simulink model "SynchronouslChange0"  (R2017b)
settings: Solver=ode23tb  StartTime=0.0  StopTime=0.5  MaxStep=1e-4  RelTol=1e-3
libraries: powerlib x7, simulink x1
settings Model: Creator=80573  LastModifiedBy=80573

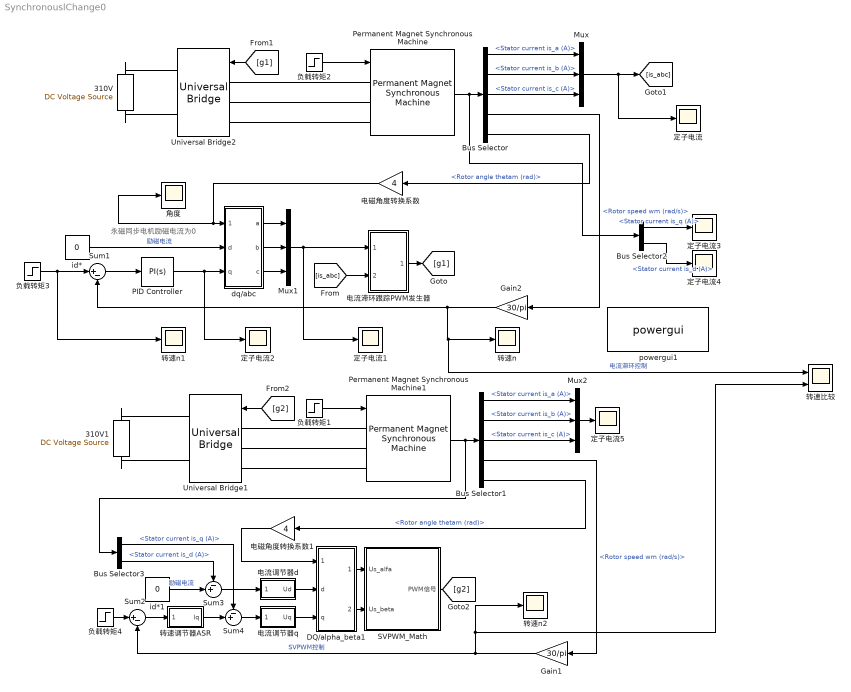
== system SynchronouslChange0 ==
  note: 永磁同步电机励磁电流为0
  310V : powerlib/Electrical Sources/DC Voltage Source  Amplitude=310  Measurements=None
  310V1 : powerlib/Electrical Sources/DC Voltage Source  Amplitude=310  Measurements=None
  Bus Selector : BusSelector  OutputSignals=Stator current is_a (A),Stator current is_b (A),Stator current is_c (A),Rotor speed wm (rad/s),Rotor angle thetam (rad)
  Bus Selector1 : BusSelector  OutputSignals=Stator current is_a (A),Stator current is_b (A),Stator current is_c (A),Rotor speed wm (rad/s),Rotor angle thetam (rad)
  Bus Selector2 : BusSelector  OutputSignals=Stator current is_q (A),Stator current is_d (A)
  Bus Selector3 : BusSelector  OutputSignals=Stator current is_q (A),Stator current is_d (A)
  DQ/alpha_beta1 : Subsystem
  Gain1 : Gain  Gain=30/pi
  Gain2 : Gain  Gain=30/pi
  Mux : Mux  Inputs=3
  Mux1 : Mux  Inputs=3
  Mux2 : Mux  Inputs=3
  PID Controller : simulink/Continuous/PID Controller  Controller=PI  TimeDomain=Continuous-time  SampleTime=-1  IntegratorMethod=Forward Euler  FilterMethod=Forward Euler  Form=Parallel  UseFilter=on  ControllerParametersSource=internal  P=0.05  I=8  D=0  N=100  InitialConditionSource=internal  InitialConditionForIntegrator=0  InitialConditionForFilter=0  ExternalReset=none  LimitOutput=on  UpperSaturationLimit=200  LowerSaturationLimit=-inf  LinearizeAsGain=on  AntiWindupMode=none  Kb=1  TrackingMode=off  Kt=1  PParamMin=[]  PParamMax=[]  IParamMin=[]  IParamMax=[]  DParamMin=[]  DParamMax=[]  NParamMin=[]  NParamMax=[]  KbParamMin=[]  KbParamMax=[]  KtParamMin=[]  KtParamMax=[]  POutMin=[]  POutMax=[]  IOutMin=[]  IOutMax=[]  DOutMin=[]  DOutMax=[]  NOutMin=[]  NOutMax=[]  KbOutMin=[]  KbOutMax=[]  KtOutMin=[]  KtOutMax=[]  IntegratorOutMin=[]  IntegratorOutMax=[]  FilterOutMin=[]  FilterOutMax=[]  SumOutMin=[]  SumOutMax=[]  SumI1OutMin=[]  SumI1OutMax=[]  SumI2OutMin=[]  SumI2OutMax=[]  SumI3OutMin=[]  SumI3OutMax=[]  SumDOutMin=[]  SumDOutMax=[]  SaturationOutMin=[]  SaturationOutMax=[]  IntegratorContinuousStateAttributes=''  IntegratorStateMustResolveToSignalObject=off  IntegratorRTWStateStorageClass=Auto  FilterContinuousStateAttributes=''  FilterStateMustResolveToSignalObject=off  FilterRTWStateStorageClass=Auto  DifferentiatorICPrevScaledInput=0  DifferentiatorOutMin=[]  DifferentiatorOutMax=[]  InitialConditionSetting=State (most efficient)  FilterDiffOutCoefMin=[]  FilterDiffOutCoefMax=[]  SumDenOutMin=[]  SumDenOutMax=[]  SumNumOutMin=[]  SumNumOutMax=[]  ReciprocalOutMin=[]  ReciprocalOutMax=[]  DivideOutMin=[]  DivideOutMax=[]  TunerSelectOption=Transfer Function Based (PID Tuner App)
  Permanent Magnet Synchronous Machine : powerlib/Machines/Permanent Magnet Synchronous Machine  NbPhases=3  FluxDistribution=Sinusoidal  RotorType=Salient-pole  MechanicalLoad=Torque Tm  PresetModel=No  ShowDetailedParameters=on  MeasurementBus=off  Resistance=2.785  Inductance=8.5e-3  dqInductances=[0.0085 0.0085]  La=0.02682  MachineConstant=Flux linkage established by magnets (V.s)  Flux=0.175  VoltageCst=126.966  TorqueCst=1.05  Flat=120  Mechanical=[0.001 0.008 4 0]  PolePairs=2  InitialConditions=[0,0, 0,0]  InitialConditions5ph=[0 0 0 0 0 0]  TsPowergui=0  TsBlock=-1  RefAngle=Aligned with phase A axis (original Park)
      settings: SourceProductName=Simscape Power Systems
  Permanent Magnet Synchronous Machine1 : powerlib/Machines/Permanent Magnet Synchronous Machine  NbPhases=3  FluxDistribution=Sinusoidal  RotorType=Salient-pole  MechanicalLoad=Torque Tm  PresetModel=No  ShowDetailedParameters=on  MeasurementBus=off  Resistance=2.785  Inductance=8.5e-3  dqInductances=[0.0085 0.0085]  La=0.02682  MachineConstant=Flux linkage established by magnets (V.s)  Flux=0.175  VoltageCst=126.966  TorqueCst=1.05  Flat=120  Mechanical=[0.001 0.008 4 0]  PolePairs=2  InitialConditions=[0,0, 0,0]  InitialConditions5ph=[0 0 0 0 0 0]  TsPowergui=0  TsBlock=-1  RefAngle=Aligned with phase A axis (original Park)
      settings: SourceProductName=Simscape Power Systems
  SVPWM_Math : Subsystem
  Sum1 : Sum  Inputs=|+-
  Sum2 : Sum  Inputs=|+-
  Sum3 : Sum  Inputs=-+|
  Sum4 : Sum  Inputs=-+|
  Universal Bridge1 : powerlib/Power Electronics/Universal Bridge  Arms=3  SnubberResistance=1e5  SnubberCapacitance=inf  Device=IGBT / Diodes  Ron=1e-3  Lon=0  ForwardVoltages="[  0  0  ]"  ForwardVoltage=0  GTOparameters=[ 10e-6 , 20e-6 ]  IGBTparameters=[ 1e-6 , 2e-6 ]  Measurements=None  Measurements_2=None  converterType=Rectifier
  Universal Bridge2 : powerlib/Power Electronics/Universal Bridge  Arms=3  SnubberResistance=1e5  SnubberCapacitance=inf  Device=IGBT / Diodes  Ron=1e-3  Lon=0  ForwardVoltages="[  0  0  ]"  ForwardVoltage=0  GTOparameters=[ 10e-6 , 20e-6 ]  IGBTparameters=[ 1e-6 , 2e-6 ]  Measurements=None  Measurements_2=None  converterType=Rectifier
  dq/abc : Subsystem
  id* : Constant  Value=0
  id*1 : Constant  Value=0
  powergui1 : powerlib/powergui  SimulationMode=Discrete  SampleTime=1e-6  frequency=50  Iterations=50  frequencyindice=0  Pbase=100e6  ErrMax=1e-4  UnitsV=kV  UnitsW=MW  buscounter=0  FunctionMessages=off  echomessages=off  EnableUseOfTLC=off  CurrentSourceSwitches=off  DisableSnubberDevices=off  DisableRonSwitches=off  DisableVfSwitches=off  DisplayEquations=off  SolverType=Tustin/Backward Euler (TBE)  Interpol=off  ExternalGateDelay=off  methode=off  Ts=100  x0status=zero  SPID=on  SwTol=0  HookPort=off  RestoreLinks=warning  ResistiveCurrentMeasurement=off  Frange=[0:2:500]  Ylog=off  Xlog=on  ShowGrid=off  save=off  variable=ZData  structure=0  ZoomFFT=on  StartTime=0.0  cycles=1  DisplayStyle=1  fundamental=60  FreqAxis=off  MaxFrequency=1000  frequencyindicesteady=1  RmsSteady=1  display=off
  定子电流{,1..5} (6 alike) : Scope
  电流滞环跟踪PWM发生器 : Subsystem
  电流调节器d : Subsystem
  电流调节器q : Subsystem
  电磁角度转换系数 : Gain  Gain=4
  电磁角度转换系数1 : Gain  Gain=4
  角度 : Scope
  负载转矩1 : Step  Time=0.2  Before=10  After=20  SampleTime=0
  负载转矩2 : Step  Time=0.2  Before=10  After=20  SampleTime=0
  负载转矩3 : Step  Time=0.3  Before=1000  After=1200  SampleTime=0
  负载转矩4 : Step  Time=0.3  Before=1000  After=1200  SampleTime=0
  转速n : Scope
  转速n1 : Scope
  转速n2 : Scope
  转速比较 : Scope  NumInputPorts=2
  转速调节器ASR : Subsystem
  wires:
  转速调节器ASR/1(Iq) -> Sum4/2
  id*/1 -> dq/abc/2(d)  "励磁电流"
  负载转矩1/1 -> Permanent Magnet Synchronous Machine1/1
  DQ/alpha_beta1/2(beta) -> SVPWM_Math/2(Us_beta)
  Bus Selector1/1 -> Mux2/1  "<Stator current is_a (A)>"
  Bus Selector1/2 -> Mux2/2  "<Stator current is_b (A)>"
  负载转矩4/1 -> Sum2/1
  电流调节器q/1(Uq) -> DQ/alpha_beta1/3(q)
  Gain1/1 -> Sum2/2, 转速比较/2, 转速n2/1  "SVPWM控制"
  Mux2/1 -> 定子电流5/1
  Permanent Magnet Synchronous Machine1/1 -> Bus Selector3/1, Bus Selector1/1
  Bus Selector3/2 -> Sum3/1  "<Stator current is_d (A)>"
  Bus Selector1/5 -> 电磁角度转换系数1/1  "<Rotor angle thetam (rad)>"
  Bus Selector2/2 -> 定子电流4/1  "<Stator current is_d (A)>"
  [g2] -> Universal Bridge1/1
  Bus Selector1/4 -> Gain1/1  "<Rotor speed wm (rad/s)>"
  Sum1/1 -> PID Controller/1
  电磁角度转换系数1/1 -> DQ/alpha_beta1/1(theta)
  Sum2/1 -> 转速调节器ASR/1("  ")
  dq/abc/2(b) -> Mux1/2
  Sum4/1 -> 电流调节器q/1("  ")
  id*1/1 -> Sum3/2  "励磁电流"
  [g1] -> Universal Bridge2/1
  电磁角度转换系数/1 -> 角度/1, dq/abc/1(theta)
  负载转矩2/1 -> Permanent Magnet Synchronous Machine/1
  Bus Selector/2 -> Mux/2  "<Stator current is_b (A)>"
  Bus Selector/3 -> Mux/3  "<Stator current is_c (A)>"
  Bus Selector3/1 -> Sum4/1  "<Stator current is_q (A)>"
  dq/abc/1(a) -> Mux1/1
  Bus Selector/5 -> 电磁角度转换系数/1  "<Rotor angle thetam (rad)>"
  负载转矩3/1 -> 转速n1/1, Sum1/1
  Permanent Magnet Synchronous Machine/1 -> Bus Selector2/1, Bus Selector/1
  Bus Selector/1 -> Mux/1  "<Stator current is_a (A)>"
  电流调节器d/1(Ud) -> DQ/alpha_beta1/2(d)
  Bus Selector2/1 -> 定子电流3/1  "<Stator current is_q (A)>"
  Bus Selector1/3 -> Mux2/3  "<Stator current is_c (A)>"
  Gain2/1 -> Sum1/2, 转速比较/1, 转速n/1  "电流滞环控制"
  DQ/alpha_beta1/1(alpha) -> SVPWM_Math/1(Us_alfa)
  [is_abc] -> 电流滞环跟踪PWM发生器/2(Iabc)
  Mux1/1 -> 电流滞环跟踪PWM发生器/1(Iabc*), 定子电流1/1
  Bus Selector/4 -> Gain2/1  "<Rotor speed wm (rad/s)>"
  Sum3/1 -> 电流调节器d/1("  ")
  dq/abc/3(c) -> Mux1/3
  Mux/1 -> 定子电流/1, [is_abc]
  SVPWM_Math/1(PWM信号) -> [g2]
  PID Controller/1 -> 定子电流2/1, dq/abc/3(q)
  电流滞环跟踪PWM发生器/1(pulse) -> [g1]
  connections:
  Universal Bridge1/LConn3 -- Permanent Magnet Synchronous Machine1/LConn3
  Universal Bridge2/LConn1 -- Permanent Magnet Synchronous Machine/LConn1
  310V/RConn1 -- Universal Bridge2/RConn1
  Universal Bridge2/LConn3 -- Permanent Magnet Synchronous Machine/LConn3
  Universal Bridge1/LConn1 -- Permanent Magnet Synchronous Machine1/LConn1
  310V/LConn1 -- Universal Bridge2/RConn2
  310V1/LConn1 -- Universal Bridge1/RConn2
  Universal Bridge1/LConn2 -- Permanent Magnet Synchronous Machine1/LConn2
  Universal Bridge2/LConn2 -- Permanent Magnet Synchronous Machine/LConn2
  310V1/RConn1 -- Universal Bridge1/RConn1

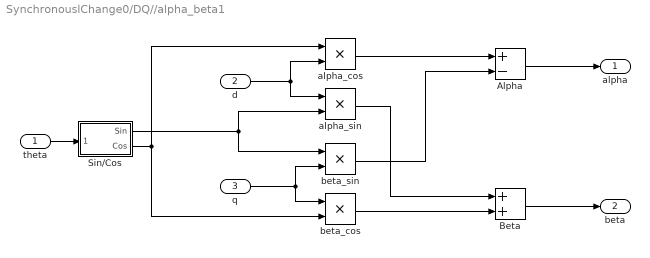
== system SynchronouslChange0/DQ//alpha_beta1 ==
  theta : Inport
  d : Inport  Port=2
  q : Inport  Port=3
  Alpha : Sum  Inputs=+-
  Beta : Sum
  Sin/Cos : Subsystem
  alpha_cos : Product
  alpha_sin : Product
  beta_cos : Product
  beta_sin : Product
  alpha : Outport
  beta : Outport  Port=2
  wires:
  Sin/Cos/2(Cos) -> beta_cos/2, alpha_cos/1
  q/1 -> beta_sin/2, beta_cos/1
  Sin/Cos/1(Sin) -> beta_sin/1, alpha_sin/2
  alpha_sin/1 -> Beta/1
  theta/1 -> Sin/Cos/1(theta)
  beta_sin/1 -> Alpha/2
  beta_cos/1 -> Beta/2
  Alpha/1 -> alpha/1
  alpha_cos/1 -> Alpha/1
  d/1 -> alpha_cos/2, alpha_sin/1
  Beta/1 -> beta/1

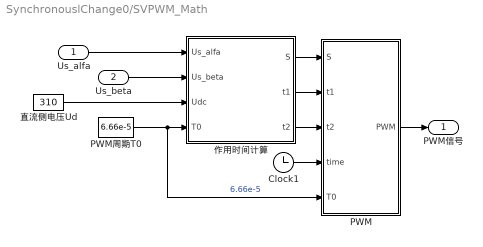
== system SynchronouslChange0/SVPWM_Math ==
  Us_alfa : Inport
  Us_beta : Inport  Port=2
  Clock1 : Clock
  PWM : MATLAB Function  TreatAsAtomicUnit=on
  PWM周期T0 : Constant  Value=6.66e-5
  作用时间计算 : MATLAB Function  TreatAsAtomicUnit=on
  直流侧电压Ud : Constant  Value=310
  PWM信号 : Outport
  wires:
  作用时间计算/2(t1) -> PWM/2(t1)
  作用时间计算/3(t2) -> PWM/3(t2)
  PWM/1(PWM) -> PWM信号/1
  Us_alfa/1 -> 作用时间计算/1(Us_alfa)
  Us_beta/1 -> 作用时间计算/2(Us_beta)
  直流侧电压Ud/1 -> 作用时间计算/3(Udc)
  PWM周期T0/1 -> PWM/5(T0), 作用时间计算/4(T0)  "6.66e-5"
  Clock1/1 -> PWM/4(time)
  作用时间计算/1(S) -> PWM/1(S)

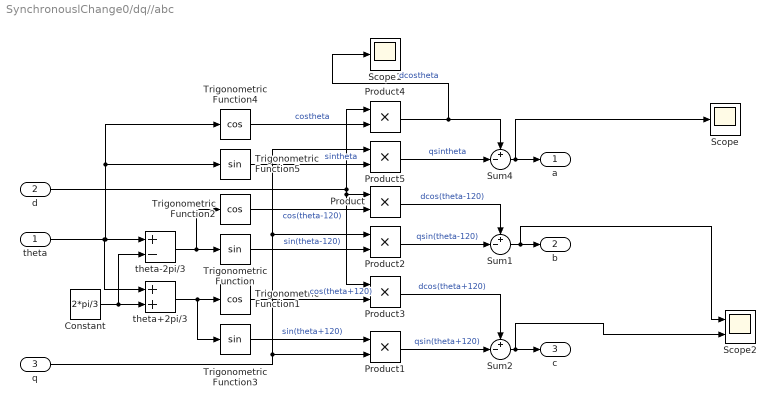
== system SynchronouslChange0/dq//abc ==
  theta : Inport
  d : Inport  Port=2
  q : Inport  Port=3
  Constant : Constant  Value=2*pi/3
  Product{,1..5} (6 alike) : Product
  Scope : Scope
  Scope1 : Scope
  Scope2 : Scope  NumInputPorts=2
  Sum1 : Sum  Inputs=+-|
  Sum2 : Sum  Inputs=+-|
  Sum4 : Sum  Inputs=+-|
  Trigonometric Function : Trigonometry
  Trigonometric Function1 : Trigonometry  Operator=cos
  Trigonometric Function2 : Trigonometry  Operator=cos
  Trigonometric Function3 : Trigonometry
  Trigonometric Function4 : Trigonometry  Operator=cos
  Trigonometric Function5 : Trigonometry
  theta+2pi/3 : Sum
  theta-2pi/3 : Sum  Inputs=+-
  a : Outport
  b : Outport  Port=2
  c : Outport  Port=3
  wires:
  Trigonometric Function5/1 -> Product5/2  "sintheta"
  Product/1 -> Sum1/1  "dcos(theta-120)"
  Trigonometric Function1/1 -> Product3/2  "cos(theta+120)"
  Product3/1 -> Sum2/1  "dcos(theta+120)"
  d/1 -> Product/1, Product3/1, Product4/1
  Constant/1 -> theta+2pi/3/2, theta-2pi/3/2
  theta/1 -> Trigonometric Function4/1, Trigonometric Function5/1, theta-2pi/3/1, theta+2pi/3/1
  theta+2pi/3/1 -> Trigonometric Function3/1, Trigonometric Function1/1
  q/1 -> Product5/1, Product2/1, Product1/2
  Trigonometric Function/1 -> Product2/2  "sin(theta-120)"
  Product4/1 -> Scope1/1, Sum4/1  "dcostheta"
  Product5/1 -> Sum4/2  "qsintheta"
  theta-2pi/3/1 -> Trigonometric Function2/1, Trigonometric Function/1
  Product1/1 -> Sum2/2  "qsin(theta+120)"
  Trigonometric Function2/1 -> Product/2  "cos(theta-120)"
  Sum4/1 -> Scope/1, a/1
  Sum1/1 -> Scope2/1, b/1
  Trigonometric Function4/1 -> Product4/2  "costheta"
  Trigonometric Function3/1 -> Product1/1  "sin(theta+120)"
  Product2/1 -> Sum1/2  "qsin(theta-120)"
  Sum2/1 -> Scope2/2, c/1

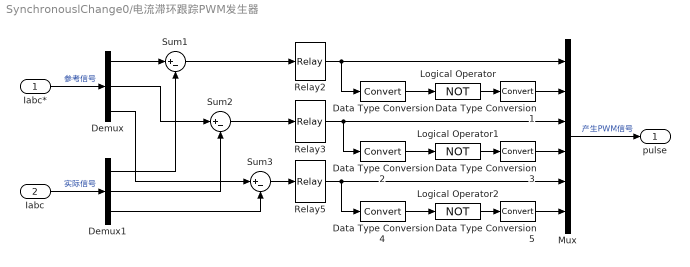
== system SynchronouslChange0/电流滞环跟踪PWM发生器 ==
  Iabc* : Inport
  Iabc : Inport  Port=2
  Data Type Conversion{,1..5} (6 alike) : DataTypeConversion
  Demux : Demux  Outputs=3
  Demux1 : Demux  Outputs=3
  Logical Operator : Logic  Operator=NOT  Inputs=1  AllPortsSameDT=off
  Logical Operator1 : Logic  Operator=NOT  Inputs=1  AllPortsSameDT=off
  Logical Operator2 : Logic  Operator=NOT  Inputs=1  AllPortsSameDT=off
  Mux : Mux  Inputs=6
  Relay2 : Relay  OnSwitchValue=0.1  OffSwitchValue=-0.1  ZeroCross=off
  Relay3 : Relay  OnSwitchValue=0.1  OffSwitchValue=-0.1  ZeroCross=off
  Relay5 : Relay  OnSwitchValue=0.1  OffSwitchValue=-0.1  ZeroCross=off
  Sum1 : Sum  Inputs=|+-
  Sum2 : Sum  Inputs=|+-
  Sum3 : Sum  Inputs=|+-
  pulse : Outport
  wires:
  Relay2/1 -> Data Type Conversion/1, Mux/1
  Data Type Conversion/1 -> Logical Operator/1
  Logical Operator/1 -> Data Type Conversion1/1
  Data Type Conversion1/1 -> Mux/2
  Mux/1 -> pulse/1  "产生PWM信号"
  Sum1/1 -> Relay2/1
  Demux/1 -> Sum1/1
  Demux1/3 -> Sum3/2
  Iabc/1 -> Demux1/1  "实际信号"
  Iabc*/1 -> Demux/1  "参考信号"
  Sum2/1 -> Relay3/1
  Logical Operator1/1 -> Data Type Conversion3/1
  Data Type Conversion3/1 -> Mux/4
  Data Type Conversion2/1 -> Logical Operator1/1
  Relay3/1 -> Data Type Conversion2/1, Mux/3
  Logical Operator2/1 -> Data Type Conversion5/1
  Data Type Conversion5/1 -> Mux/6
  Data Type Conversion4/1 -> Logical Operator2/1
  Relay5/1 -> Data Type Conversion4/1, Mux/5
  Sum3/1 -> Relay5/1
  Demux/2 -> Sum2/1
  Demux1/1 -> Sum1/2
  Demux1/2 -> Sum2/2
  Demux/3 -> Sum3/1

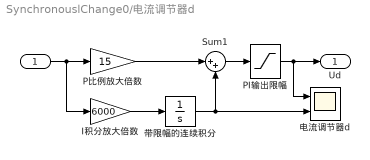
== system SynchronouslChange0/电流调节器d ==
  "  " : Inport
  I积分放大倍数 : Gain  Gain=6000
  PI输出限幅 : Saturate  UpperLimit=400  LowerLimit=-400
  P比例放大倍数 : Gain  Gain=15
  Sum1 : Sum  Inputs=|++
  带限幅的连续积分 : Integrator  UpperSaturationLimit=30  LowerSaturationLimit=-30
  电流调节器d : Scope  NumInputPorts=2
  Ud : Outport
  wires:
  Sum1/1 -> PI输出限幅/1
  PI输出限幅/1 -> 电流调节器d/1, Ud/1
  P比例放大倍数/1 -> Sum1/1
  I积分放大倍数/1 -> 带限幅的连续积分/1
  带限幅的连续积分/1 -> 电流调节器d/2, Sum1/2
  "  "/1 -> I积分放大倍数/1, P比例放大倍数/1

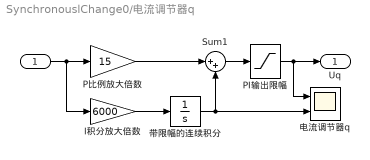
== system SynchronouslChange0/电流调节器q ==
  "  " : Inport
  I积分放大倍数 : Gain  Gain=6000
  PI输出限幅 : Saturate  UpperLimit=300  LowerLimit=-300
  P比例放大倍数 : Gain  Gain=15
  Sum1 : Sum  Inputs=|++
  带限幅的连续积分 : Integrator  LimitOutput=on  UpperSaturationLimit=400  LowerSaturationLimit=-400
  电流调节器q : Scope  NumInputPorts=2
  Uq : Outport
  wires:
  Sum1/1 -> PI输出限幅/1
  PI输出限幅/1 -> 电流调节器q/1, Uq/1
  P比例放大倍数/1 -> Sum1/1
  I积分放大倍数/1 -> 带限幅的连续积分/1
  带限幅的连续积分/1 -> 电流调节器q/2, Sum1/2
  "  "/1 -> I积分放大倍数/1, P比例放大倍数/1

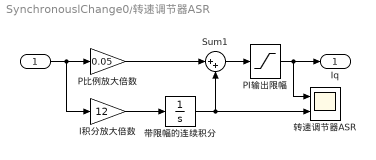
== system SynchronouslChange0/转速调节器ASR ==
  "  " : Inport
  I积分放大倍数 : Gain  Gain=12
  PI输出限幅 : Saturate  UpperLimit=25  LowerLimit=-25
  P比例放大倍数 : Gain  Gain=0.05
  Sum1 : Sum  Inputs=|++
  带限幅的连续积分 : Integrator  LimitOutput=on  UpperSaturationLimit=30  LowerSaturationLimit=-30
  转速调节器ASR : Scope  NumInputPorts=2
  Iq : Outport
  wires:
  Sum1/1 -> PI输出限幅/1
  PI输出限幅/1 -> 转速调节器ASR/1, Iq/1
  P比例放大倍数/1 -> Sum1/1
  I积分放大倍数/1 -> 带限幅的连续积分/1
  带限幅的连续积分/1 -> 转速调节器ASR/2, Sum1/2
  "  "/1 -> I积分放大倍数/1, P比例放大倍数/1

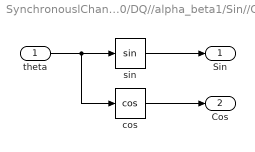
== system SynchronouslChange0/DQ//alpha_beta1/Sin//Cos ==
  theta : Inport
  cos : Trigonometry  Operator=cos
  sin : Trigonometry
  Sin : Outport
  Cos : Outport  Port=2
  wires:
  sin/1 -> Sin/1
  theta/1 -> sin/1, cos/1
  cos/1 -> Cos/1

== matlab function SynchronouslChange0/SVPWM_Math/作用时间计算 ==
  data: Us_alfa input; S output; Us_beta input; Udc input; T0 input; t1 output; t2 output
function [S,t1,t2] = fcn(Us_alfa,Us_beta,Udc,T0)
% This block supports an embeddable subset of the MATLAB language.
% See the help menu for details.
%--------------------为了方便推导作用时间做出的设定值------------------------
X=sqrt(3)*T0*Us_beta/Udc;                           
Y=sqrt(3)/2*T0*Us_beta/Udc+3/2*T0*Us_alfa/Udc;     
Z=sqrt(3)/2*T0*Us_beta/Udc-3/2*T0*Us_alfa/Udc;      
%--------------------------------扇区值判断---------------------------------
%Uref1*sqrt(3)
%(Uref1+Uref2)*sqrt(3)
%(Uref1+Uref3)*sqrt(3)
%--------------------------------------------------------------------------
if(Us_beta>0)                                       %Uref1>0
    A=1;
else
    A=0;
end                                                                                                                                                                                                                                                                                                                                                                                                                                                                                                                                                                                                                                                                                                                                                                                                                                                                                                                                                                                                                                                                                                                                                                                                                                                                                   
if((sqrt(3)*Us_alfa-Us_beta)>0)                     %Uref2>0
    B=1;
else
    B=0; 
end
if((-sqrt(3)*Us_alfa-Us_beta)>0)                    %%Uref3>0
    C=1;
else
    C=0;
end
N=A+2*B+4*C;                                        %扇区值N，而不是扇区编号！！！！！！！
%--------------------------------------------------------------------------
%-----------------------------------分割线----------------------------------

%-----------------------------矢量作用时间计算-------------------------------
%--------------------------------S为扇区编号-------------------------------
switch(N)
    case 1
        S=2;%----------------------扇区编号S---------------------------
        t1=Z; 
        t2=Y; 
    case 2
        S=6;
        t1=Y; 
        t2=-X;
    case 3
        S=1;
        t1=-Z; 
        t2=X;
    case 4
        S=4;
        t1=-X; 
        t2=Z;
    case 5
        S=3;
        t1=X; 
        t2=-Y;
    case 6
        S=5;
        t1=-Y; 
        t2=-Z;
    otherwise
        S=1;
        t1=0; 
        t2=0;        
end
%--------------------------------------------------------------------------
%-----------------------------是否需要调制判断------------------------------
if((t1+t2)>T0)
    t11=t1*T0/(t1+t2);
    t21=t2*T0/(t1+t2);
    t1=t11;
    t2=t21;
    t0=0;
else
t0=T0-t1-t2;
end
%--------------------------------------------------------------------------

== matlab function SynchronouslChange0/SVPWM_Math/PWM ==
  data: S input double; PWM output double size=[1 6]; t1 input double; t2 input double; time input double; T0 input double
function PWM =fcn(S,t1,t2,time,T0)
% This block supports an embeddable subset of the MATLAB language.
% See the help menu for details. 
%------------------------------普通定义电压---------------------------------
%U0=[0 0 0];U1=[1 0 0];U2=[1 1 0];U3=[0 1 0];
%U4=[0 1 1];U5=[0 0 1];U6=[1 0 1];U7=[1 1 1];
%------------------------由上可得八种电压输出信号控制（每种后面取反）---------
U0=[0 1 0 1 0 1];U1=[1 0 0 1 0 1];U2=[1 0 1 0 0 1];U3=[0 1 1 0 0 1];
U4=[0 1 1 0 1 0];U5=[0 1 0 1 1 0];U6=[1 0 0 1 1 0];U7=[1 0 1 0 1 0];
%----------------------------此处采用二进制定义电压--------------------------
%U0=[0 0 0];U1=[0 0 1];U2=[0 1 0];U3=[0 1 1];
%U4=[1 0 0];U5=[1 0 1];U6=[1 1 0];U7=[1 1 1];
%------------------------由上可得八种电压输出信号控制（每种后面取反）---------
%U0=[0 1 0 1 0 1];U1=[0 1 0 1 1 0];U2=[0 1 1 0 0 1];U3=[0 1 1 0 1 0];
%U4=[1 0 0 1 0 1];U5=[1 0 0 1 1 0];U6=[1 0 1 0 0 1];U7=[1 0 1 0 1 0];
%--------------------------------------------------------------------------
%----------------------为了方便确定扇区切换时间设定的Tx、Ty、Tz---------------
t0=T0-t1-t2;
Ta=t0/4;
Tb=Ta+t1/2;
Tc=Tb+t2/2;
t=rem(time,T0);%t=时间time/周期Ts的余数 即在每个周期内作用的时间轴时间t
G=U0;
%------------------------------扇区编号S------------------------------------
%-------------------------------分割线--------------------------------------
switch (S)
    case 1
        G1=U1;
        G2=U2;
    case 2
        G1=U3;
        G2=U2;
    case 3
        G1=U3;
        G2=U4;
    case 4
        G1=U5;
        G2=U4;
    case 5
        G1=U5;
        G2=U6;
    case 6
        G1=U1;
        G2=U6;
    otherwise
        G1=U0;
        G2=U7;
end
%---------------------------七步分量法--------------------------------------
if (t<Ta)
	G=U0;       
elseif((t>=Ta)&&(t<Tb))
    G=G1;
elseif((t>=Tb)&&(t<Tc))
    G=G2;
elseif((t>=Tc)&&(t<(T0-Tc)))
    G=U7;
elseif((t>=(T0-Tc))&&(t<(T0-Tb)))
    G=G2;
elseif((t>=(T0-Tb))&&(t<(T0-Ta)))
    G=G1;
elseif((t>=(T0-Ta))&&(t<T0))
    G=U0;
end
PWM=G;
end
